simulink model "CoolingFanWithFaults"  (R2023b)
settings: Solver=FixedStepAuto  StartTime=0.0  StopTime=SimEndTime  FixedStep=0.1  RelTol=1e-3
model workspace (MAT data in the model file):
  ConvectionFanPowerMax = 5
  ConvectionFanPowerMin = 0
  ConvectionFanPowerStartTime = 0
  ConvectionFanPowerTimeMin = 86400
  CoolingFanOutputTopic = 'tempcoolingfan'
  DCSourceNumAnomalies = 4
  DCSourceVoltageDrop = 3
  DCSourceVoltageDropDuration = 60
  DCSourceVoltageNominal = 12
  DragCoeffNominal = 8e-08
  DragIncreaseAmplitude = 8e-07
  DragIncreaseDuration = 60
  DragNoiseVariance = 10
  DragNumAnomalies = 4
  ExternalTempIncreaseAmplitude = 30
  ExternalTempIncreaseDuration = 60
  ExternalTempNumAnomalies = 4
  RngSeed = 0
  SimEndTime = 86400
  ThermalHeatCoeffMax = 1000
  ThermalHeatCoeffMin = 1
  ThermalHeatCoeffStartTime = 0
  ThermalHeatCoeffTimeMin = 86400
undefined symbols (not defined in the file or in its folder): Subsystem, VaryingConvectionLib
libraries: fl_lib x24, nesl_utility x9, fl_ps_legacy_lib x6, ee_lib x4, AnomalyGeneratorLib x3, simulink x2
settings Model: PacingRate=2  Creator=astother  LastModifiedBy=anarasim
settings SolverCC: AlgebraicLoopSolver=TrustRegion
settings DataIOCC: LoggingToFile=on  DatasetSignalFormat=timetable  LoggingFileName=/home/anarasim/Documents/MATLAB/ExampleManager/anarasim.Bdoc23b_Examples_v2/predmaint-ex62086719/Data/CoolingFanWithFaults_log_1.mat
settings DebuggingCC: UnconnectedInputMsg=warning  UnconnectedOutputMsg=warning  UnconnectedLineMsg=warning
settings ModelReferenceCC: EnableRefExpFcnMdlSchedulingChecks=on
settings RTWCC: DLArmComputeVersion=19.05

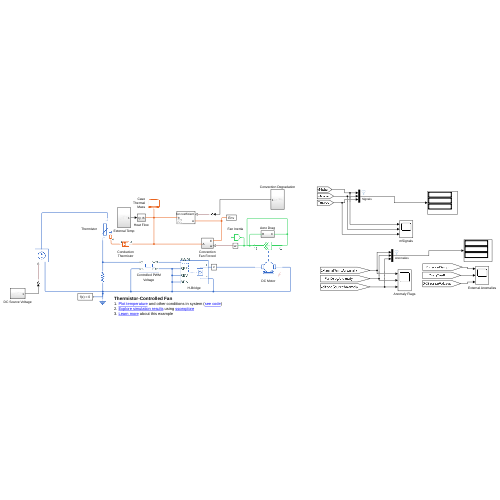
[thumbnail: Simulink's stored preview of the top-level diagram]
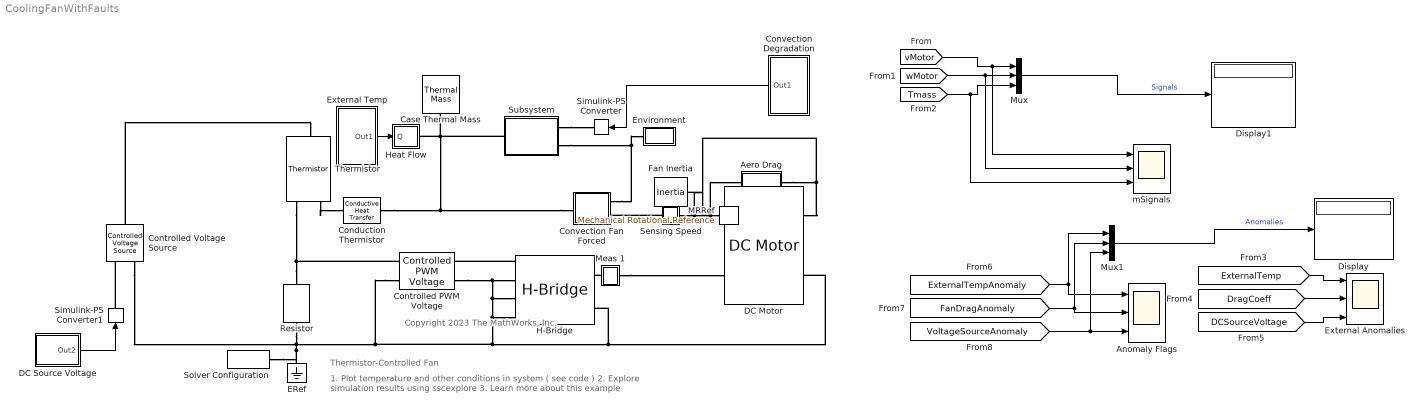
== system CoolingFanWithFaults ==
  note: Thermistor-Controlled Fan
  note: 1. Plot temperature and other conditions in system ( see code )
      | 2. Explore simulation results using sscexplore
      | 3. Learn more about this example
  note: Copyright 2023 The MathWorks, Inc.
  Aero Drag : Subsystem
  Anomaly Flags : Scope  NumInputPorts=3
  Case Thermal Mass : fl_lib/Thermal/Thermal Elements/Thermal Mass  mass_type=foundation.enum.constant_variable.constant  mass=0.1 kg  sp_heat=100 J/kg/K  mass_min=1e-6 kg  num_ports=foundation.enum.numPorts2.one  m_specify=off  m_priority=High  m=1 kg  m_nominal_specify=off  m_nominal_unit=kg  m_nominal_value=1  T_specify=on  T_priority=High  T=298.15 K  T_nominal_specify=off  T_nominal_unit=K  T_nominal_value=1  Q_specify=off  Q_priority=High  Q=0 J/s  Q_nominal_specify=off  Q_nominal_unit=J/s  Q_nominal_value=1
  Conduction Thermistor : fl_lib/Thermal/Thermal Elements/Conductive Heat Transfer  thermal_type=foundation.enum.ConstantVariableTabulated.Constant  wall_geometry=foundation.enum.ConductionWallGeometry.Planar  area=1 cm^2  thickness=1 mm  d_in=0.05 m  d_out=0.1 m  L=1 m  th_cond_min=10 W/(K*m)  th_cond=40 W/(m*K)  th_cond_TLU=[413, 401, 392, 383, 371, 357, 342] W/(K*m)  temp_TLU=[200, 273, 400, 600, 800, 1000, 1200] K  T_specify=off  T_priority=High  T=0 K  T_nominal_specify=off  T_nominal_unit=K  T_nominal_value=1  Q_specify=off  Q_priority=High  Q=0 J/s  Q_nominal_specify=off  Q_nominal_unit=J/s  Q_nominal_value=1
  Controlled PWM Voltage : ee_lib/Integrated Circuits/Controlled PWM Voltage  F=1000 Hz  TD=0 s  pulse_width_offset=0 s  pulse_min=0 s  pwm_or_av=2  event_type=1  sample_time=1e-6 s  Vmin=0 V  Vmax=12 V  Vm=5 V  u_min=0  u_max=1
  Controlled Voltage Source : fl_lib/Electrical/Electrical Sources/Controlled Voltage Source
  Convection Fan Forced : Subsystem
  Convection Degradation : Subsystem
  DC Motor : ee_lib/Electromechanical/Brushed Motors/DC Motor  field_option=ee.enum.field_option.pm  Rf=100 Ohm  Lf=1 H  Laf=0.15 H  If0=0 A  parameterization=ee.enum.dcparam_option.load_speed  Ra=0.3 Ohm  La=1e-04 H  emf_or_torque=ee.enum.emf_or_torque.kv  Kv=15e-04 V/rpm  Ki=6.876e-04 N*m/A  T_stall=2.4e-04 N*m  w_max=7000 rpm  w_rated=4000 rpm  P_rated=2 W  V_rated=10 V  lam_param=ee.enum.lam_param.damping  i_noload=0 A  V_i_noload=1.5 V  J=1e-6 kg*m^2  lam=1e-08 N*m/(rad/s)  speed0=0 rpm  enable_fault_armature=simscape.enum.onoff.off  rev_faulted=2 / 3  G_faulted_armature=1e-5 S  fault_trigger_armature=ee.enum.faults.faultTrigger.temporal  t_fault_armature=20 s  max_permissible_current_armature=inf A  t_fail_on_current_armature=1 s  enable_fault_field=simscape.enum.onoff.off  G_faulted_field=1e-5 S  fault_trigger_field=ee.enum.faults.faultTrigger.temporal  t_fault_field=1 s  max_permissible_current_field=inf A  t_fail_on_current_field=1 s  fault_action=simscape.enum.assert.action.none  alpha=3.93e-3 1/K  Tmeas=25 degC  thermal_mass=100 J/K  initial_temperature=25 degC
  DC Source Voltage : Subsystem
  Display : Display
  Display1 : Display
  ERef : fl_lib/Electrical/Electrical Elements/Electrical Reference
  Environment : Subsystem
      mask Display: disp('Env')
  External Anomalies : Scope  NumInputPorts=3
  External Temp : Subsystem
  Fan Inertia : fl_lib/Mechanical/Rotational Elements/Inertia  inertia=1e-5 kg*m^2  num_ports=foundation.enum.numPorts2.one  w_specify=on  w_priority=High  w=0 rad/s  w_nominal_specify=off  w_nominal_unit=rad/s  w_nominal_value=1  t_specify=off  t_priority=High  t=0 N*m  t_nominal_specify=off  t_nominal_unit=N*m  t_nominal_value=1
  H-Bridge : ee_lib/Semiconductors & Converters/Converters/H-Bridge  supply_ports=ee.enum.supply_ports.hidesupply  pwm_or_av=2  regenerative_braking_mode=2  discontinuous=0  freewheeling_mode=1  Rload=10 Ohm  Lload=1e-5 H  F=10 kHz  Venable=2.5 V  Vmax=5 V  Vreverse=2.5 V  Vbrake=2.5 V  Vm=12 V  Ron=0.1 Ohm  Don=0.1 Ohm  Goff=1e-6 S  Tmeas=298.15 K  Ron2=0.1 Ohm  Don2=0.05 Ohm  Tmeas2=398.15 K  thermal_mass=100 J/K  initial_temperature=298.15 K
  Heat Flow : Subsystem
  MRRef : fl_lib/Mechanical/Rotational Elements/Mechanical Rotational Reference
  Meas 1 : Subsystem
      mask Display: disp('v')
  Mux : Mux  Inputs=3
  Mux1 : Mux  Inputs=3
  Resistor : fl_lib/Electrical/Electrical Elements/Resistor  R=100 Ohm  i_specify=off  i_priority=High  i=0 A  i_nominal_specify=off  i_nominal_unit=A  i_nominal_value=1  v_specify=off  v_priority=High  v=0 V  v_nominal_specify=off  v_nominal_unit=V  v_nominal_value=1
  Sensing Speed : Subsystem
      mask Display: disp('w')
  Simulink-PS Converter : nesl_utility/Simulink-PS Converter  PhysicalDomain=network_engine_domain  SubClassName=ps_input  LeftPortType=input  RightPortType=output  PseudoPeriodic=off  Frequencies=[]  NoiseDistribution=none  NoiseParameters=[]  Unit=1  AffineConversion=off  FilteringAndDerivatives=provide  SimscapeFilterOrder=1  InputFilterTimeConstant=0.001  UdotUserProvided=0
  Simulink-PS Converter1 : nesl_utility/Simulink-PS Converter  PhysicalDomain=network_engine_domain  SubClassName=ps_input  LeftPortType=input  RightPortType=output  PseudoPeriodic=off  Frequencies=[]  NoiseDistribution=none  NoiseParameters=[]  Unit=1  AffineConversion=off  FilteringAndDerivatives=provide  SimscapeFilterOrder=1  InputFilterTimeConstant=0.001  UdotUserProvided=0
  Solver Configuration : nesl_utility/Solver Configuration  PhysicalDomain=network_engine_domain  SubClassName=solver  LeftPortType=input  RightPortType=generic  Tones=[]  Harmonics=[]  SimulateNoise=off  Profile=off  UseLocalSampling=off  EnableSwitchedLinearOptims=on  FrequencyDomain=off  UseCCode=off  RelTol=0.001  AbsTol=1e-06  MinStep=1e-09  ToWorkspace=off  RevertToSquareIcSolve=off  NumHomotopyIterations=100  PhasorMode=off  PhasorModeNumHarmonics=1  ConsistencySolver=NEWTON_FTOL  IndexReductionMethod=DerivativeReplacement  DoDC=off  ResidualTolerance=1e-9  ConsistencyTolSource=GLOBAL  ConsistencyAbsTol=0.001  ConsistencyRelTol=0.001  ConsistencyTolFactor=0.001  UseLocalSolver=off  LocalSolverChoice=NE_BACKWARD_EULER_ADVANCER  ResolveIndetEquations=on  FunctionEvalNumThread=1  LocalSolverSampleTime=.001  DoFixedCost=off  MaxNonlinIter=3  MaxModeIter=2  ComputeImpulses=off  ImpulseIterations=2  LinearAlgebra=auto  LinearAlgebraNumThread=0  EquationFormulation=NE_TIME_EF  DelaysMemoryBudget=1024  AutomaticFiltering=on  FilteringTimeConstant=0.001  PartitionStorageMethod=AS_NEEDED  PartitionMemoryBudget=1024  PartitionMethod=FAST  MultibodyUseLocalSolver=off  MultibodyLocalSolverChoice=ODE1  MultibodyLocalSolverSampleTime=0.001
  Subsystem : Subsystem  AncestorBlock=VaryingConvectionLib/Subsystem
      settings: LibrarySourceBlock=VaryingConvectionLib/Subsystem
  Thermistor : ee_lib/Sensors & Transducers/Thermistor  R0=1000 Ohm  Bparam=3.5e+04 K  T0=25 degC  tc=5 s  K_d=7.5e-04 W/K  T_specify=on  T_priority=High  T=25 degC  T_nominal_specify=off  T_nominal_unit=K  T_nominal_value=1
      settings: InternalSimscapePortConfiguration="{\"Bottom\":[],\"Left\":[{\"id\":\"A\",\"label\":\"A\",\"type\":\"foundation.thermal.thermal\"},{\"id\":\"p\",\"label\":\"+\",\"type\":\"foundation.electrical.electrical\"}],\"Right\":[{\"id\":\"n\",\"label\":\"-\",\"type\":\"foundation.electrical.electrical\"}],\"Top\":[]}"
  mSignals : Scope  NumInputPorts=3
  wires:
  [Tmass] -> mSignals/3, Mux/3
  [ExternalTempAnomaly] -> Mux1/1, Anomaly Flags/1
  [VoltageSourceAnomaly] -> Mux1/3, Anomaly Flags/3
  Mux/1 -> Display1/1  "Signals"
  [vMotor] -> mSignals/1, Mux/1
  [DCSourceVoltage] -> External Anomalies/3
  External Temp/1(Out1) -> Heat Flow/1(Q)
  Convection Degradation/1(Out1) -> Simulink-PS Converter/1
  [DragCoeff] -> External Anomalies/2
  Mux1/1 -> Display/1  "Anomalies"
  [ExternalTemp] -> External Anomalies/1
  DC Source Voltage/1(Out2) -> Simulink-PS Converter1/1
  [wMotor] -> mSignals/2, Mux/2
  [FanDragAnomaly] -> Mux1/2, Anomaly Flags/2
  connections:
  Convection Fan Forced/LConn1 -- Conduction Thermistor/LConn1 -- Subsystem/RConn1 -- Case Thermal Mass/LConn1 -- Heat Flow/RConn1
  Controlled PWM Voltage/LConn2 -- Controlled PWM Voltage/RConn2 -- H-Bridge/LConn2 -- H-Bridge/LConn3 -- H-Bridge/LConn4 -- H-Bridge/RConn2 -- DC Motor/RConn1 -- Controlled Voltage Source/RConn2 -- Resistor/RConn1 -- ERef/LConn1 -- Solver Configuration/RConn1
  MRRef/LConn1 -- Aero Drag/RConn1 -- DC Motor/RConn2
  Fan Inertia/LConn1 -- Sensing Speed/LConn1 -- Aero Drag/LConn1 -- DC Motor/LConn2
  Resistor/LConn1 -- Controlled PWM Voltage/LConn1 -- Thermistor/LConn2
  Environment/LConn1 -- Convection Fan Forced/RConn1 -- Subsystem/LConn2
  Subsystem/LConn1 -- Simulink-PS Converter/RConn1
  Controlled Voltage Source/LConn1 -- Thermistor/RConn1
  Meas 1/RConn1 -- H-Bridge/RConn1
  Meas 1/LConn1 -- DC Motor/LConn1
  Thermistor/LConn1 -- Conduction Thermistor/RConn1
  H-Bridge/LConn1 -- Controlled PWM Voltage/RConn1
  Sensing Speed/RConn1 -- Convection Fan Forced/RConn2
  Simulink-PS Converter1/RConn1 -- Controlled Voltage Source/RConn1

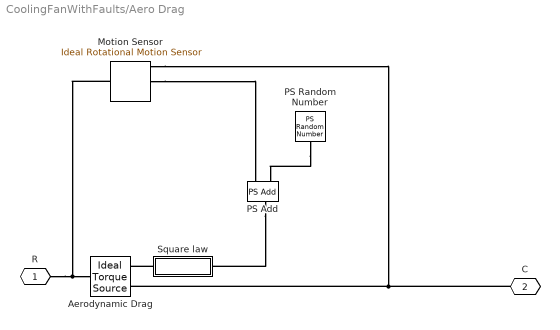
== system CoolingFanWithFaults/Aero Drag ==
  Aerodynamic Drag : fl_lib/Mechanical/Mechanical Sources/Ideal Torque Source
  Motion Sensor : fl_lib/Mechanical/Mechanical Sensors/Ideal Rotational Motion Sensor  reference=foundation.enum.MeasurementReference.difference  acceleration_port=false  velocity_port=true  position_port=true  wrap_angle=simscape.enum.onoff.off  offset=0 deg
  PS Add : fl_ps_legacy_lib/Legacy Physical Signals/Functions/PS Add
      settings: InternalSimscapePortConfiguration="{\"Bottom\":[],\"Left\":[{\"id\":\"I1\",\"label\":\"\",\"type\":\"input\"},{\"id\":\"I2\",\"label\":\"\",\"type\":\"input\"}],\"Right\":[{\"id\":\"O\",\"label\":\"\",\"type\":\"output\"}],\"Top\":[]}"
  PS Random Number : fl_lib/Physical Signals/Sources/PS Random Number  mean=0  variance=DragNoiseVariance  initial_seed=0  sample_time=0.1 s
      settings: InternalSimscapePortConfiguration="{\"Bottom\":[],\"Left\":[],\"Right\":[{\"id\":\"Y\",\"label\":\"Y\",\"type\":\"output\"}],\"Top\":[]}"
  Square law : Subsystem
  R : PMIOPort  Side=Left
  C : PMIOPort  Port=2  Side=Right
  connections:
  R/RConn1 -- Motion Sensor/LConn1 -- Aerodynamic Drag/LConn1
  C/RConn1 -- Aerodynamic Drag/RConn2 -- Motion Sensor/RConn1
  Square law/RConn1 -- Aerodynamic Drag/RConn1
  Motion Sensor/RConn2 -- PS Add/LConn2
  PS Add/RConn1 -- Square law/LConn1
  PS Random Number/RConn1 -- PS Add/LConn1

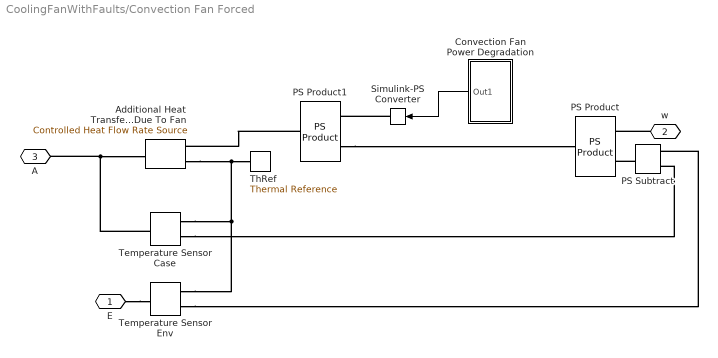
== system CoolingFanWithFaults/Convection Fan Forced ==
  Additional Heat Transfer Due To Fan : fl_lib/Thermal/Thermal Sources/Controlled Heat Flow Rate Source
  Convection Fan Power Degradation : Subsystem
  PS Product : fl_ps_legacy_lib/Legacy Physical Signals/Functions/PS Product
  PS Product1 : fl_ps_legacy_lib/Legacy Physical Signals/Functions/PS Product
  PS Subtract : fl_ps_legacy_lib/Legacy Physical Signals/Functions/PS Subtract
  Simulink-PS Converter : nesl_utility/Simulink-PS Converter  PhysicalDomain=network_engine_domain  SubClassName=ps_input  LeftPortType=input  RightPortType=output  PseudoPeriodic=off  Frequencies=[]  NoiseDistribution=none  NoiseParameters=[]  Unit=1  AffineConversion=off  FilteringAndDerivatives=provide  SimscapeFilterOrder=1  InputFilterTimeConstant=0.001  UdotUserProvided=0
  Temperature Sensor Case : fl_lib/Thermal/Thermal Sensors/Temperature Sensor  temperature_measure=foundation.enum.MeasurementReference.difference
  Temperature Sensor Env : fl_lib/Thermal/Thermal Sensors/Temperature Sensor  temperature_measure=foundation.enum.MeasurementReference.difference
  ThRef : fl_lib/Thermal/Thermal Elements/Thermal Reference
  E : PMIOPort  Side=Right
  w : PMIOPort  Port=2  Side=Right
  A : PMIOPort  Port=3  Side=Left
  wires:
  Convection Fan Power Degradation/1(Out1) -> Simulink-PS Converter/1
  connections:
  Temperature Sensor Case/LConn1 -- A/RConn1 -- Additional Heat Transfer Due To Fan/LConn1
  Temperature Sensor Case/RConn2 -- PS Subtract/LConn2
  Temperature Sensor Case/RConn1 -- Temperature Sensor Env/RConn1 -- Additional Heat Transfer Due To Fan/RConn2 -- ThRef/LConn1
  PS Subtract/RConn1 -- PS Product/LConn2
  w/RConn1 -- PS Product/LConn1
  PS Product1/LConn2 -- PS Product/RConn1
  PS Product1/RConn1 -- Additional Heat Transfer Due To Fan/RConn1
  Temperature Sensor Env/RConn2 -- PS Subtract/LConn1
  E/RConn1 -- Temperature Sensor Env/LConn1
  Simulink-PS Converter/RConn1 -- PS Product1/LConn1

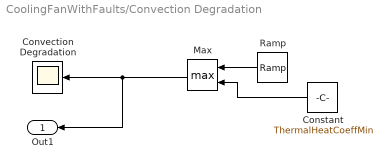
== system CoolingFanWithFaults/Convection Degradation ==
  Constant : Constant  Value=ThermalHeatCoeffMin  VectorParams1D=off  SampleTime=-1
  Convection Degradation : Scope
  Max : MinMax  Function=max  Inputs=2
  Ramp : simulink/Sources/Ramp  slope=-(ThermalHeatCoeffMax-ThermalHeatCoeffMin)/ThermalHeatCoeffTimeMin  start=ThermalHeatCoeffStartTime  InitialOutput=ThermalHeatCoeffMax
  Out1 : Outport
  wires:
  Constant/1 -> Max/2
  Ramp/1 -> Max/1
  Max/1 -> Convection Degradation/1, Out1/1

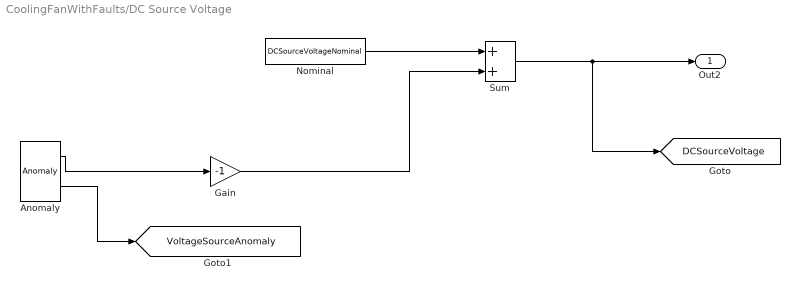
== system CoolingFanWithFaults/DC Source Voltage ==
  Anomaly : AnomalyGeneratorLib/Anomaly  EndTime=SimEndTime  NumAnomalies=DCSourceNumAnomalies  AnomalyDuration=DCSourceVoltageDropDuration  AnomalyAmplitude=DCSourceVoltageDrop  RngSeed=RngSeed
  Gain : Gain  Gain=-1
  Nominal : Constant  Value=DCSourceVoltageNominal
  Sum : Sum
  Out2 : Outport
  tag scope: DCSourceVoltage=global, VoltageSourceAnomaly=global
  wires:
  Nominal/1 -> Sum/1
  Anomaly/1 -> Gain/1
  Sum/1 -> Out2/1, [DCSourceVoltage]
  Gain/1 -> Sum/2
  Anomaly/2 -> [VoltageSourceAnomaly]

== system CoolingFanWithFaults/Environment ==
  Air Temperature : fl_lib/Physical Signals/Sources/PS Constant  constant=298.15
  Temperature Source : fl_lib/Thermal/Thermal Sources/Controlled Temperature Source
  ThRef : fl_lib/Thermal/Thermal Elements/Thermal Reference
  B : PMIOPort  Side=Left
  connections:
  Air Temperature/RConn1 -- Temperature Source/RConn1
  ThRef/LConn1 -- Temperature Source/RConn2
  B/RConn1 -- Temperature Source/LConn1

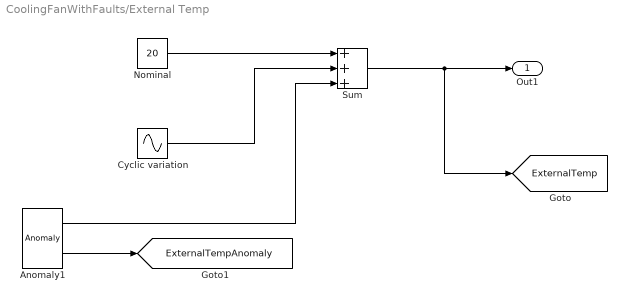
== system CoolingFanWithFaults/External Temp ==
  Anomaly1 : AnomalyGeneratorLib/Anomaly  EndTime=SimEndTime  NumAnomalies=ExternalTempNumAnomalies  AnomalyDuration=ExternalTempIncreaseDuration  AnomalyAmplitude=ExternalTempIncreaseAmplitude  RngSeed=RngSeed+2
  Cyclic variation : Sin  Amplitude=2  Frequency=2*pi/(60*60*24)  SampleTime=0
  Nominal : Constant  Value=20
  Sum : Sum  Inputs=+++
  Out1 : Outport
  tag scope: ExternalTemp=global, ExternalTempAnomaly=global
  wires:
  Nominal/1 -> Sum/1
  Cyclic variation/1 -> Sum/2
  Sum/1 -> [ExternalTemp], Out1/1
  Anomaly1/1 -> Sum/3
  Anomaly1/2 -> [ExternalTempAnomaly]

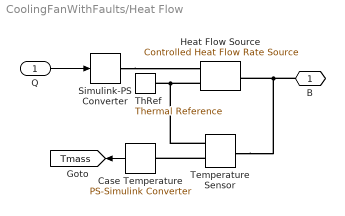
== system CoolingFanWithFaults/Heat Flow ==
  Q : Inport
  Case Temperature : nesl_utility/PS-Simulink Converter  PhysicalDomain=network_engine_domain  SubClassName=ps_output  LeftPortType=input  RightPortType=output  PseudoPeriodic=off  Frequencies=[]  VectorFormat=1-D array  Unit=degC  AffineConversion=on
  Heat Flow Source : fl_lib/Thermal/Thermal Sources/Controlled Heat Flow Rate Source
  Simulink-PS Converter : nesl_utility/Simulink-PS Converter  PhysicalDomain=network_engine_domain  SubClassName=ps_input  LeftPortType=input  RightPortType=output  PseudoPeriodic=off  Frequencies=[]  NoiseDistribution=none  NoiseParameters=[]  Unit=1  AffineConversion=off  FilteringAndDerivatives=zero  SimscapeFilterOrder=1  InputFilterTimeConstant=.001  UdotUserProvided=0
  Temperature Sensor : fl_lib/Thermal/Thermal Sensors/Temperature Sensor  temperature_measure=foundation.enum.MeasurementReference.difference
  ThRef : fl_lib/Thermal/Thermal Elements/Thermal Reference
  B : PMIOPort  Side=Right
  tag scope: Tmass=global
  wires:
  Q/1 -> Simulink-PS Converter/1
  Case Temperature/1 -> [Tmass]
  connections:
  Heat Flow Source/RConn2 -- Temperature Sensor/RConn1 -- ThRef/LConn1
  Simulink-PS Converter/RConn1 -- Heat Flow Source/RConn1
  B/RConn1 -- Temperature Sensor/LConn1 -- Heat Flow Source/LConn1
  Temperature Sensor/RConn2 -- Case Temperature/LConn1

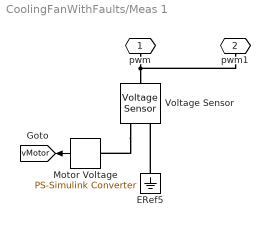
== system CoolingFanWithFaults/Meas 1 ==
  ERef5 : fl_lib/Electrical/Electrical Elements/Electrical Reference
  Motor Voltage : nesl_utility/PS-Simulink Converter  PhysicalDomain=network_engine_domain  SubClassName=ps_output  LeftPortType=input  RightPortType=output  PseudoPeriodic=off  Frequencies=[]  VectorFormat=1-D array  Unit=V  AffineConversion=off
  Voltage Sensor : fl_lib/Electrical/Electrical Sensors/Voltage Sensor
  pwm : PMIOPort  Side=Left
  pwm1 : PMIOPort  Port=2  Side=Right
  tag scope: vMotor=global
  wires:
  Motor Voltage/1 -> [vMotor]
  connections:
  Voltage Sensor/LConn1 -- pwm/RConn1 -- pwm1/RConn1
  ERef5/LConn1 -- Voltage Sensor/RConn2
  Voltage Sensor/RConn1 -- Motor Voltage/LConn1

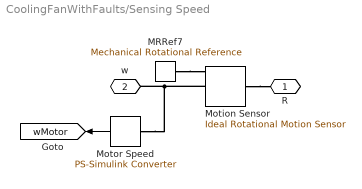
== system CoolingFanWithFaults/Sensing Speed ==
  MRRef7 : fl_lib/Mechanical/Rotational Elements/Mechanical Rotational Reference
  Motion Sensor : fl_lib/Mechanical/Mechanical Sensors/Ideal Rotational Motion Sensor  reference=foundation.enum.MeasurementReference.difference  acceleration_port=false  velocity_port=true  position_port=true  wrap_angle=simscape.enum.onoff.off  offset=0 deg
  Motor Speed : nesl_utility/PS-Simulink Converter  PhysicalDomain=network_engine_domain  SubClassName=ps_output  LeftPortType=input  RightPortType=output  PseudoPeriodic=off  Frequencies=[]  VectorFormat=1-D array  Unit=rpm  AffineConversion=off
  R : PMIOPort  Side=Left
  w : PMIOPort  Port=2  Side=Right
  tag scope: wMotor=global
  wires:
  Motor Speed/1 -> [wMotor]
  connections:
  Motion Sensor/LConn1 -- R/RConn1
  Motion Sensor/RConn2 -- Motor Speed/LConn1 -- w/RConn1
  MRRef7/LConn1 -- Motion Sensor/RConn1

== system CoolingFanWithFaults/Subsystem ==
  Varying convection transfer : SimscapeComponentBlock  SourceFile=convection_with_heat_coeff_input  ComponentPath=convection_with_heat_coeff_input  ComponentVariants="[\"convection_with_heat_coeff_input\"]"  ComponentVariantNames="[\"convection_with_heat_coeff_input\"]"  ClassName=convection_with_heat_coeff_input  SchemaVersion=1  area=1e-4 m^2  T_specify=off  T_priority=None  T=0 K  T_nominal_specify=off  T_nominal_unit=K  T_nominal_value=1  Q_specify=off  Q_priority=None  Q=0 W  Q_nominal_specify=off  Q_nominal_unit=W  Q_nominal_value=1
      settings: CopyFcn=simscape.engine.sli.internal.componentblockcallback(gcbh,'COPY')  PreCopyFcn=simscape.engine.sli.internal.componentblockcallback(gcbh,'PRECOPY')  PreDeleteFcn=simscape.engine.sli.internal.componentblockcallback(gcbh,'PREDELETE')  InternalSimscapePortConfiguration="{\"Bottom\":[],\"Left\":[{\"id\":\"A\",\"label\":\"A\",\"type\":\"foundation.thermal.thermal\"},{\"id\":\"heat_tr_coeff\",\"label\":\"Heat transfer coefficient\",\"type\":\"input\"}],\"Right\":[{\"id\":\"B\",\"label\":\"B\",\"type\":\"foundation.thermal.thermal\"}],\"Top\":[]}"
      mask Type: Convective Heat Transfer
  Heat transfer coefficient : PMIOPort  Side=Left
  B : PMIOPort  Port=2  Side=Right
  A : PMIOPort  Port=3  Side=Left
  connections:
  Varying convection transfer/LConn2 -- Heat transfer coefficient/RConn1
  Varying convection transfer/RConn1 -- B/RConn1
  Varying convection transfer/LConn1 -- A/RConn1

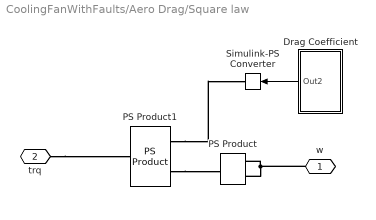
== system CoolingFanWithFaults/Aero Drag/Square law ==
  Drag Coefficient : Subsystem
  PS Product : fl_ps_legacy_lib/Legacy Physical Signals/Functions/PS Product
  PS Product1 : fl_ps_legacy_lib/Legacy Physical Signals/Functions/PS Product
  Simulink-PS Converter : nesl_utility/Simulink-PS Converter  PhysicalDomain=network_engine_domain  SubClassName=ps_input  LeftPortType=input  RightPortType=output  PseudoPeriodic=off  Frequencies=[]  NoiseDistribution=none  NoiseParameters=[]  Unit=1  AffineConversion=off  FilteringAndDerivatives=provide  SimscapeFilterOrder=1  InputFilterTimeConstant=0.001  UdotUserProvided=0
  w : PMIOPort  Side=Left
  trq : PMIOPort  Port=2  Side=Right
  wires:
  Drag Coefficient/1(Out2) -> Simulink-PS Converter/1
  connections:
  w/RConn1 -- PS Product/LConn2 -- PS Product/LConn1
  trq/RConn1 -- PS Product1/RConn1
  PS Product1/LConn2 -- PS Product/RConn1
  PS Product1/LConn1 -- Simulink-PS Converter/RConn1

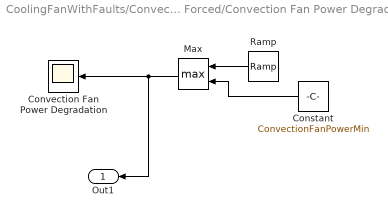
== system CoolingFanWithFaults/Convection Fan Forced/Convection Fan Power Degradation ==
  Constant : Constant  Value=ConvectionFanPowerMin  VectorParams1D=off  SampleTime=-1
  Convection Fan Power Degradation : Scope
  Max : MinMax  Function=max  Inputs=2
  Ramp : simulink/Sources/Ramp  slope=-(ConvectionFanPowerMax-ConvectionFanPowerMin)/ConvectionFanPowerTimeMin  start=ConvectionFanPowerStartTime  InitialOutput=ConvectionFanPowerMax
  Out1 : Outport
  wires:
  Ramp/1 -> Max/1
  Max/1 -> Out1/1, Convection Fan Power Degradation/1
  Constant/1 -> Max/2

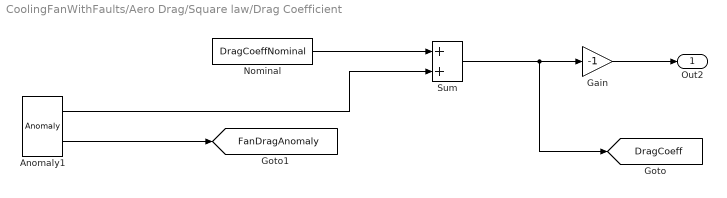
== system CoolingFanWithFaults/Aero Drag/Square law/Drag Coefficient ==
  Anomaly1 : AnomalyGeneratorLib/Anomaly  EndTime=SimEndTime  NumAnomalies=DragNumAnomalies  AnomalyDuration=DragIncreaseDuration  AnomalyAmplitude=DragIncreaseAmplitude  RngSeed=RngSeed+1
  Gain : Gain  Gain=-1
  Nominal : Constant  Value=DragCoeffNominal
  Sum : Sum
  Out2 : Outport
  tag scope: DragCoeff=global, FanDragAnomaly=global
  wires:
  Sum/1 -> [DragCoeff], Gain/1
  Nominal/1 -> Sum/1
  Anomaly1/1 -> Sum/2
  Gain/1 -> Out2/1
  Anomaly1/2 -> [FanDragAnomaly]
